simulink model "visualization"  (R2019a)
settings: Solver=VariableStepAuto  StartTime=0.0  StopTime=50  RelTol=1e-3
libraries: aerolibanim x1
settings Model: EnablePacing=on  Creator=Gaming  LastModifiedBy=Gaming

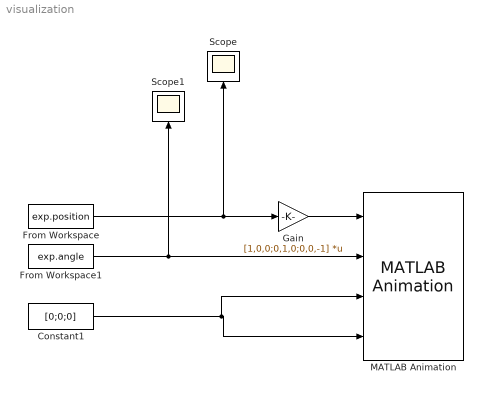
== system visualization ==
  Constant1 : Constant  Value=[0;0;0]
  From Workspace : FromWorkspace  VariableName=exp.position  SampleTime=0
  From Workspace1 : FromWorkspace  VariableName=exp.angle  SampleTime=0
  Gain : Gain  Gain=[1,0,0;0,1,0;0,0,-1]  Multiplication=Matrix(K*u)
  MATLAB Animation : aerolibanim/MATLAB Animation  Tag=Matlab Animation 6 DOF  Vehicles=2  Geometries={'astredwedge.mat','floor.ac'}  BoundingBoxCoordinates=[-50,50,-50,50,-50,50]  CameraOffset=[-110,-90,-10]  CameraViewAngle=3  SampleTime=0.03  FigurePosition=[1,41,1920,990]
      settings: SourceProductName=Aerospace Blockset  SourceProductBaseCode=AE
  Scope : Scope
  Scope1 : Scope
  wires:
  From Workspace/1 -> Gain/1, Scope/1
  Constant1/1 -> MATLAB Animation/3, MATLAB Animation/4
  Gain/1 -> MATLAB Animation/1
  From Workspace1/1 -> Scope1/1, MATLAB Animation/2
